simulink model "q5"  (R2024b)
settings: Solver=ode4  StartTime=0.0  StopTime=TF  FixedStep=DT  RelTol=1e-3
values from neighbouring files (symbols this model uses):
  U0 = [0.525841853692 -0.00469375602825 0 0 0]    [ICs_aircraft2_180Kts_CG1.mat]    (also in ICs_aircraft2_180Kts_CG2.mat = [0.525939752377 -0.00596702425354 0 0 0]; ICs_aircraft2_75Kts_CG1.mat = [0.0938327586982 -0.025121721174 0 0 0]; ICs_aircraft2_75Kts_CG2.mat = [0.0933937108451 -0.0325384431522 0 0 0])
  X0 = [92.595040743 0 0.87765052501 0 0 0 0 0.00947809123249 0 0 0 -91.44]    [ICs_aircraft2_180Kts_CG1.mat]    (also in ICs_aircraft2_180Kts_CG2.mat = [92.5949054744 0 0.891807618371 0 0 0 0 0.00963098390968 0 0; ICs_aircraft2_75Kts_CG1.mat = [38.2773569622 0 4.84683742125 0 0 0 0 0.125953827189 0 0 0 ; ICs_aircraft2_75Kts_CG2.mat = [38.2730356766 0 4.88084307236 0 0 0 0 0.126842278514 0 0 0 )
undefined symbols (not defined in the file or in its folder): A, B, C, D, FlightData, Xg
settings Model: Creator=Boyang  LastModifiedBy=Kaitlyn
settings DataIOCC: SaveState=on
settings OptimizationCC: ReuseModelBlockBuffer=off
settings RTWCC: GPUComputeCapability=3.5

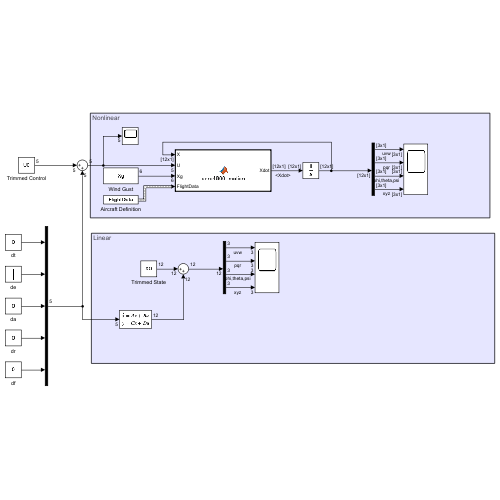
[thumbnail: Simulink's stored preview of the top-level diagram]
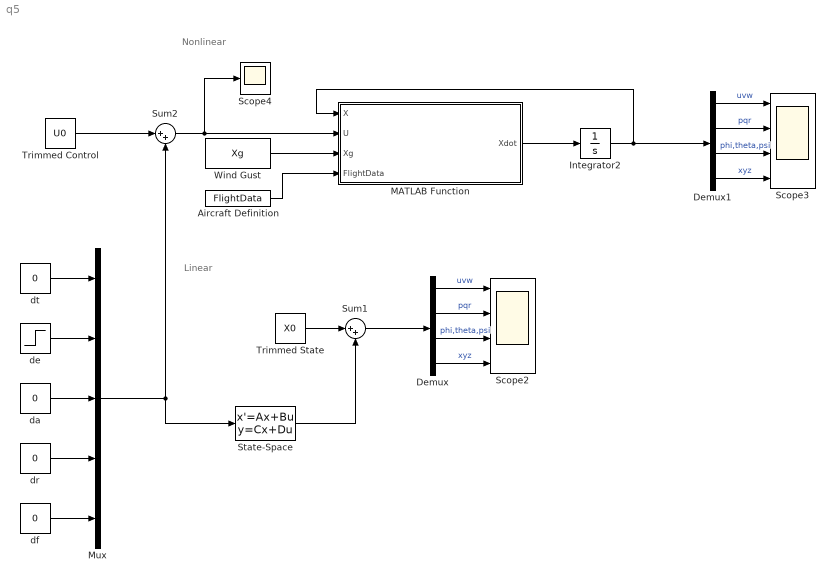
== system q5 ==
  note: Linear
  note: Nonlinear
  Aircraft Definition : Constant  Value=FlightData  OutDataTypeStr=Bus:FD_bus
  Demux : Demux
  Demux1 : Demux
  Integrator2 : Integrator  InitialCondition=X0
  MATLAB Function : MATLAB Function  TreatAsAtomicUnit=on
  Mux : Mux  Inputs=5
  Scope2 : Scope  NumInputPorts=4
  Scope3 : Scope  NumInputPorts=4
  Scope4 : Scope
  State-Space : StateSpace  A=A  B=B  C=C  D=D  InitialCondition=0  ContinuousStateAttributes={'u', 'v', 'w', 'p', 'q', 'r', 'phi', 'theta', 'psi', 'x', 'y', 'z'}
  Sum1 : Sum  Inputs=|++
  Sum2 : Sum  Inputs=|++
  Trimmed Control : Constant  Value=U0
  Trimmed State : Constant  Value=X0
  Wind Gust : Constant  Value=Xg
  da : Constant  Value=0
  de : Step  Time=10  After=1*pi/180  SampleTime=0
  df : Constant  Value=0
  dr : Constant  Value=0
  dt : Constant  Value=0
  wires:
  dt/1 -> Mux/1
  de/1 -> Mux/2
  da/1 -> Mux/3
  dr/1 -> Mux/4
  df/1 -> Mux/5
  Mux/1 -> State-Space/1, Sum2/2
  Trimmed State/1 -> Sum1/1
  State-Space/1 -> Sum1/2
  Demux/1 -> Scope2/1  "uvw"
  Demux/2 -> Scope2/2  "pqr"
  Demux/3 -> Scope2/3  "phi,theta,psi"
  Demux/4 -> Scope2/4  "xyz"
  MATLAB Function/1(Xdot) -> Integrator2/1
  Trimmed Control/1 -> Sum2/1
  Sum2/1 -> MATLAB Function/2(U), Scope4/1
  Wind Gust/1 -> MATLAB Function/3(Xg)
  Demux1/4 -> Scope3/4  "xyz"
  Demux1/3 -> Scope3/3  "phi,theta,psi"
  Demux1/2 -> Scope3/2  "pqr"
  Demux1/1 -> Scope3/1  "uvw"
  Integrator2/1 -> MATLAB Function/1(X), Demux1/1
  Aircraft Definition/1 -> MATLAB Function/4(FlightData)
  Sum1/1 -> Demux/1

== matlab function q5/MATLAB Function ==
  data: X input; Xdot output; U input; Xg input; FlightData input
function Xdot = aero4600_motion(X, U, Xg, FlightData)

% Calculate Airpath Properties
Vt = sqrt((X(1)+Xg(1))^2 + (X(2)+Xg(2))^2 + (X(3)+Xg(3))^2);
alpha = atan((X(3)+Xg(3))/(X(1)+Xg(1)));
beta  = asin((X(2)+Xg(2))/Vt);

% Calculate Atmosphere Properties
[ rho, ~ ] = aero4600_atmos(-X(12,1));
qbar = 0.5*rho*Vt^2;

% Normalised Parameters
bo2V   = 0.5*FlightData.Geo.b/Vt;
co2V   = 0.5*FlightData.Geo.c/Vt;
%da_a = (Xdot(3)/X(1)-X(3)*Xdot(1)*X(1)^-2)*co2V;
%db_a = (Xdot(2)/X(1)-X(2)*Xdot(1)*X(1)^-2)*bo2V;
p_a  = (X(4)+Xg(4))*bo2V;
q_a  = (X(5)+Xg(5))*co2V;
r_a  = (X(6)+Xg(6))*bo2V;

% Lift/Drag Force Coefficients
sig = rho/1.2256;
C_t = (FlightData.Prop.P_max*(1.1324*sig-0.1324)*FlightData.Prop.eta*U(1)/Vt)/qbar/FlightData.Geo.S;   % As an X-wise force coefficient
CL = FlightData.Aero.CLo + FlightData.Aero.CLa*alpha;
Cd = FlightData.Aero.Cdo + FlightData.Aero.k*CL^2;

% Force Coefficients
Sa = sin(alpha);
Ca = cos(alpha);
Cx = -Cd*Ca + CL*Sa + C_t;
Cx_x3dot = 0;
Cx_x2dot = 0;
Cx_x1dot = 0;

%Cy =  FlightData.Aero.Cyb*beta + FlightData.Aero.Cybd*db_a + FlightData.Aero.Cyp*p_a + FlightData.Aero.Cyr*r_a + FlightData.Aero.Cyda*U(3) + FlightData.Aero.Cydr*U(4) ;
Cy =  FlightData.Aero.Cyb*beta + FlightData.Aero.Cyp*p_a + FlightData.Aero.Cyr*r_a + FlightData.Aero.Cyda*U(3) + FlightData.Aero.Cydr*U(4) ;
Cy_x3dot = 0;
Cy_x2dot = bo2V*FlightData.Aero.Cybd/X(1);
Cy_x1dot = -bo2V*FlightData.Aero.Cybd*X(2)/(X(1)^2);

%Cz = -CL*Ca - Cd*Sa - FlightData.Aero.CLad*da_a - FlightData.Aero.CLq*q_a - FlightData.Aero.CLde*U(2) - FlightData.Aero.CLdf*U(5);
Cz = -CL*Ca - Cd*Sa - FlightData.Aero.CLq*q_a - FlightData.Aero.CLde*U(2) - FlightData.Aero.CLdf*U(5);
Cz_x3dot = -co2V*FlightData.Aero.CLad/X(1);
Cz_x2dot = 0;
Cz_x1dot = co2V*FlightData.Aero.CLad*X(3)/(X(1)^2);

ForceCoeff = [Cx;Cy;Cz];


% Moment Coefficients
%Cl = FlightData.Aero.Clb*beta + FlightData.Aero.Clbd*db_a + FlightData.Aero.Clp*p_a + FlightData.Aero.Clr*r_a + FlightData.Aero.Clda*U(3) + FlightData.Aero.Cldr*U(4) ;
Cl = FlightData.Aero.Clb*beta + FlightData.Aero.Clp*p_a + FlightData.Aero.Clr*r_a + FlightData.Aero.Clda*U(3) + FlightData.Aero.Cldr*U(4) ;
Cl_x3dot = 0;
Cl_x2dot = bo2V*FlightData.Aero.Clbd/X(1);
Cl_x1dot = -bo2V*FlightData.Aero.Clbd*X(2)/(X(1)^2);

%Cm = FlightData.Aero.Cmo + FlightData.Aero.Cma*alpha + FlightData.Aero.Cmad*da_a + FlightData.Aero.Cmq*q_a + FlightData.Aero.Cmde*U(2) + FlightData.Aero.Cmdf*U(5) ;
Cm = FlightData.Aero.Cmo + FlightData.Aero.Cma*alpha + FlightData.Aero.Cmq*q_a + FlightData.Aero.Cmde*U(2) + FlightData.Aero.Cmdf*U(5) ;
Cm_x3dot = co2V*FlightData.Aero.Cmad/X(1);
Cm_x2dot = 0;
Cm_x1dot = -co2V*FlightData.Aero.Cmad*X(3)/(X(1)^2);


%Cn = FlightData.Aero.Cnb*beta + FlightData.Aero.Cnbd*db_a + FlightData.Aero.Cnp*p_a + FlightData.Aero.Cnr*r_a + FlightData.Aero.Cnda*U(3) + FlightData.Aero.Cndr*U(4) ;
Cn = FlightData.Aero.Cnb*beta + FlightData.Aero.Cnp*p_a + FlightData.Aero.Cnr*r_a + FlightData.Aero.Cnda*U(3) + FlightData.Aero.Cndr*U(4) ;
Cn_x3dot = 0;
Cn_x2dot = bo2V*FlightData.Aero.Cnbd/X(1);
Cn_x1dot = -bo2V*FlightData.Aero.Cnbd*X(2)/(X(1)^2);

MomentCoeff = [Cl;Cm;Cn];


% Calculate Forces and Moments
F_x = qbar*FlightData.Geo.S*ForceCoeff(1);
F_x_3 = qbar*FlightData.Geo.S*Cx_x3dot;
F_x_2 = qbar*FlightData.Geo.S*Cx_x2dot;
F_x_1 = qbar*FlightData.Geo.S*Cx_x1dot;


F_y = qbar*FlightData.Geo.S*ForceCoeff(2);
F_y_3 = qbar*FlightData.Geo.S*Cy_x3dot;
F_y_2 = qbar*FlightData.Geo.S*Cy_x2dot;
F_y_1 = qbar*FlightData.Geo.S*Cy_x1dot;

F_z = qbar*FlightData.Geo.S*ForceCoeff(3);
F_z_3 = qbar*FlightData.Geo.S*Cz_x3dot;
F_z_2 = qbar*FlightData.Geo.S*Cz_x2dot;
F_z_1 = qbar*FlightData.Geo.S*Cz_x1dot;

M_x = qbar*FlightData.Geo.S*FlightData.Geo.b*MomentCoeff(1);
M_x_3 = qbar*FlightData.Geo.S*FlightData.Geo.b*Cl_x3dot;
M_x_2 = qbar*FlightData.Geo.S*FlightData.Geo.b*Cl_x2dot;
M_x_1 = qbar*FlightData.Geo.S*FlightData.Geo.b*Cl_x1dot;

M_y = qbar*FlightData.Geo.S*FlightData.Geo.c*MomentCoeff(2);
M_y_3 = qbar*FlightData.Geo.S*FlightData.Geo.c*Cm_x3dot;
M_y_2 = qbar*FlightData.Geo.S*FlightData.Geo.c*Cm_x2dot;
M_y_1 = qbar*FlightData.Geo.S*FlightData.Geo.c*Cm_x1dot;


M_z = qbar*FlightData.Geo.S*FlightData.Geo.b*MomentCoeff(3);
M_z_3 = qbar*FlightData.Geo.S*FlightData.Geo.b*Cn_x3dot;
M_z_2 = qbar*FlightData.Geo.S*FlightData.Geo.b*Cn_x2dot;
M_z_1 = qbar*FlightData.Geo.S*FlightData.Geo.b*Cn_x1dot;

% Calculate Linear Acceleration
Xdot = zeros(12,1);
Xdot(1,1)=-FlightData.I.g*sin(X(8)) + X(6)*X(2) - X(5)*X(3) + F_x/FlightData.I.m ;
Xdot(2,1)= FlightData.I.g*sin(X(7))*cos(X(8)) - X(6)*X(1) + X(4)*X(3) + F_y/FlightData.I.m ;
Xdot(3,1)= FlightData.I.g*cos(X(7))*cos(X(8)) + X(5)*X(1) - X(4)*X(2) + F_z/FlightData.I.m ;

H = eye(12);
H(1,1) = H(1,1) - F_x_1/FlightData.I.m;
H(1,2) = H(1,2) - F_x_2/FlightData.I.m;
H(1,3) = H(1,3) - F_x_3/FlightData.I.m;
H(2,1) = H(2,1) - F_y_1/FlightData.I.m;
H(2,2) = H(2,2) - F_y_2/FlightData.I.m;
H(2,3) = H(2,3) - F_y_3/FlightData.I.m;
H(3,1) = H(3,1) - F_z_1/FlightData.I.m;
H(3,2) = H(3,2) - F_z_2/FlightData.I.m;
H(3,3) = H(3,3) - F_z_3/FlightData.I.m;


% Calculate Inertial Coefficients
c0=FlightData.I.Ixx*FlightData.I.Izz-FlightData.I.Ixz^2;
c1=FlightData.I.Izz/c0;
c2=FlightData.I.Ixz/c0;
c3=c2*(FlightData.I.Ixx-FlightData.I.Iyy+FlightData.I.Izz);
c4=c1*(FlightData.I.Iyy-FlightData.I.Izz)-c2*FlightData.I.Ixz;
c5=1/FlightData.I.Iyy;
c6=c5*FlightData.I.Ixz;
c7=c5*(FlightData.I.Izz-FlightData.I.Ixx);
c8=FlightData.I.Ixx/c0;
c9=c8*(FlightData.I.Ixx-FlightData.I.Iyy)+c2*FlightData.I.Ixz;

% Calculate Rotation Acceleration
Xdot(4,1) = c3*X(4)*X(5) + c4*X(5)*X(6) + c1*M_x + c2*M_z;
Xdot(5,1) = c7*X(4)*X(6) - c6*(X(4)^2-X(6)^2) + c5*M_y;
Xdot(6,1) = c9*X(4)*X(5) - c3*X(5)*X(6) + c2*M_x + c8*M_z;

H(4,1) = H(4,1) - c1*M_x_1 - c2*M_z_1;
H(4,2) = H(4,2) - c1*M_x_2 - c2*M_z_2;
H(4,3) = H(4,3) - c1*M_x_3 - c2*M_z_3;
H(5,1) = H(5,1) - c5*M_y_1;
H(5,2) = H(5,2) - c5*M_y_2;
H(5,3) = H(5,3) - c5*M_y_3;
H(6,1) = H(6,1) - c2*M_x_1 - c8*M_z_1;
H(6,2) = H(6,2) - c2*M_x_2 - c8*M_z_2;
H(6,3) = H(6,3) - c2*M_x_3 - c8*M_z_3;


% Calculate Euler Rates
Xdot(7,1) = X(4) + X(5)*sin(X(7))*tan(X(8)) + X(6)*cos(X(7))*tan(X(8));
Xdot(8,1) = X(5)*cos(X(7)) - X(6)*sin(X(7));
Xdot(9,1) = X(5)*sin(X(7))*sec(X(8)) + X(6)*cos(X(7))*sec(X(8));

% Calculate Lbe
lbe=[ cos(X(9))*cos(X(8)) cos(X(9))*sin(X(8))*sin(X(7))-sin(X(9))*cos(X(7)) cos(X(9))*sin(X(8))*cos(X(7))+sin(X(9))*sin(X(7))
    sin(X(9))*cos(X(8)) sin(X(9))*sin(X(8))*sin(X(7))+cos(X(9))*cos(X(7)) sin(X(9))*sin(X(8))*cos(X(7))-cos(X(9))*sin(X(7))
    -sin(X(8)) cos(X(8))*sin(X(7)) cos(X(8))*cos(X(7))];

% Calculate Position Rates
Xdot(10:12,1)=lbe*[X(1) X(2) X(3)]';

Xdot = H\Xdot;

end


function [rho,a]=aero4600_atmos(alt)
% Function to compute ambient air density and speed of sound
%
% (c) Peter W. Gibbens & S. Dumble, 1 March, 2011.
%
% Altitude in meters

lap_rate= 0.0065;   % (C)deg/meter
t0=15;            % (C)deg
rho0=1.225;         % Kg/m^3
p0=101310;          % Pa


if alt>= 11000
    temp=-56.4;
    pres=p0*(0.2189*(exp(9.81*(11000-alt)/(287.1*(temp+273)))));
    rho= rho0*(0.2972*(exp(9.81*(11000-alt)/(287.1*(temp+273)))));
else
    temp=(t0-(alt*lap_rate));
    pres=p0*((((temp+273)/(t0+273))^(9.81/(lap_rate*287.1))));
    rho =rho0*((((temp+273)/(t0+273))^((9.81-(lap_rate*287.1))/(lap_rate*287.1))));
end

a=(1.4*287.1*(temp+273))^0.5;
end
